simulink model "Trajectory_closest_point_info_get"  (R2021a)
settings: configuration reference "AION_IDS_Speedgoat" (kept outside this file)
undefined symbols (not defined in the file): CLOSEST_DISTANCE_THRESHOLD, DEG2RAD, DELTA_ANGLE_COMPENSATION1, DELTA_ANGLE_COMPENSATION2, DELTA_ANGLE_DIVISOR360, DELTA_ANGLE_THRESHOLD, N_ALTERNATIVE_CLOSEST_POINT_QUEUE, SINGLE_STEP_MOTION_ARC_LENGTH_THRESHOLD
libraries: simulink x7
(part 1 of 2)
Description:
  | 获取参考轨迹中的最近点信息
settings Model: DataDictionary=Trajectory_Closest_Point_Info_Get.sldd  Creator=xinrui  LastModifiedBy=Administrator
settings ConfigSetRef: SourceName=AION_IDS_Speedgoat

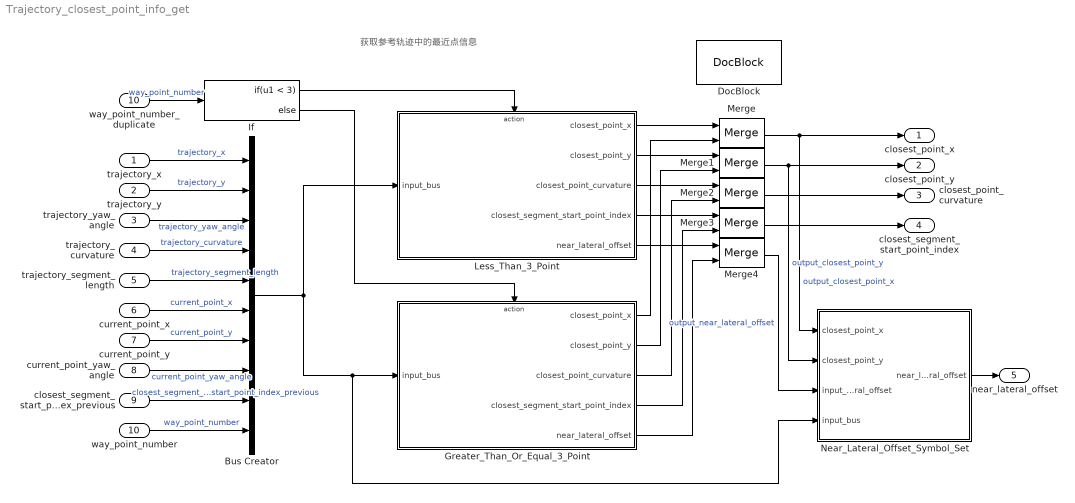
== system Trajectory_closest_point_info_get ==
  note: 获取参考轨迹中的最近点信息
  trajectory_x : Inport  Description=参考轨迹的x坐标序列，实数，m。  OutDataTypeStr=double  PortDimensions=MAX_GLOBAL_TRAJECTORY_WAY_POINT_NUMBER  Interpolate=off
  trajectory_y : Inport  Description=参考轨迹的y坐标序列，实数，m。  Port=2  OutDataTypeStr=double  PortDimensions=MAX_GLOBAL_TRAJECTORY_WAY_POINT_NUMBER  Interpolate=off
  trajectory_yaw_angle : Inport  Description=参考轨迹横摆角序列，实数，deg。  Port=3  OutDataTypeStr=double  PortDimensions=MAX_GLOBAL_TRAJECTORY_WAY_POINT_NUMBER  Interpolate=off
  trajectory_curvature : Inport  Description=参考轨迹曲率序列，实数，1/m。  Port=4  OutDataTypeStr=double  PortDimensions=MAX_GLOBAL_TRAJECTORY_WAY_POINT_NUMBER  Interpolate=off
  trajectory_segment_length : Inport  Description=参考轨迹相邻两点之间的线段长度序列，实数，m。  Port=5  OutDataTypeStr=double  PortDimensions=MAX_GLOBAL_TRAJECTORY_WAY_POINT_NUMBER  Interpolate=off
  current_point_x : Inport  Description=车辆所处的当前点x坐标，实数，m。  Port=6  OutDataTypeStr=double  Interpolate=off
  current_point_y : Inport  Description=车辆所处的当前点y坐标，实数，m。  Port=7  OutDataTypeStr=double  Interpolate=off
  current_point_yaw_angle : Inport  Description=当前车辆横摆角，实数，deg。  Port=8  OutDataTypeStr=double  Interpolate=off
  closest_segment_start_point_index_previous : Inport  Description=上周期最近路点线段起始点索引（从1开始计数），自然数，无量纲。  Port=9  OutDataTypeStr=int32  Interpolate=off
  way_point_number : Inport  Description=参考轨迹路点数量，自然数，无量纲。  Port=10  OutDataTypeStr=int32  Interpolate=off
  Bus Creator : BusCreator  Inputs=10
  DocBlock : simulink/Model-Wide Utilities/DocBlock  DocumentType=HTML  mask(DocBlock){}
      mask Display:
      | plot([.8 0 0 1 1 .8 .8 1],[1 1 0 0 .8 1 .8 .8]);
      | text(.5,.6,'CHANGELOG','horizontalalignment','center');
      | text(.95,.05,get_param(gcb,'DocumentType'),'verticalalignment','bottom','horizontalalignment','right');
  Greater_Than_Or_Equal_3_Point : Subsystem  Description=参考轨迹路点数大于等于3个时，采用局部搜索或者全局搜索获取最近点。  TreatAsAtomicUnit=on
  If : If  Description=|  IfExpression=u1 < 3
      | （1）参考轨迹路点数少于3个时使用倒数2个点进行向量投影，获取最近点。
      | （2）参考轨迹路点数大于等于3个时，采用局部搜索或者全局搜索获取最近点。
  Less_Than_3_Point : Subsystem  Description=参考轨迹路点数少于3个时使用倒数2个点进行向量投影，获取最近点。  TreatAsAtomicUnit=on
  Merge{,1..4} (5 alike) : Merge
  Near_Lateral_Offset_Symbol_Set : Subsystem  Description=设置最近处横向偏差的正负符号。
  way_point_number_duplicate : InportShadow  Description=第二个点的x坐标。  Port=10  OutDataTypeStr=int32  Interpolate=off
  closest_point_x : Outport  Description=最近点x坐标，实数，m。  OutDataTypeStr=double
  closest_point_y : Outport  Description=最近点y坐标，实数，m。  Port=2  OutDataTypeStr=double
  closest_point_curvature : Outport  Description=最近点曲率，实数，1/m。  Port=3  OutDataTypeStr=double
  closest_segment_start_point_index : Outport  Description=最近路点线段起始点索引（从1开始计数），自然数，无量纲。  Port=4  OutDataTypeStr=int32
  near_lateral_offset : Outport  Description=最近处横向偏差，实数，m。  Port=5  OutDataTypeStr=double
  wires:
  trajectory_x/1 -> Bus Creator/1  "trajectory_x"
  trajectory_y/1 -> Bus Creator/2  "trajectory_y"
  trajectory_yaw_angle/1 -> Bus Creator/3  "trajectory_yaw_angle"
  trajectory_curvature/1 -> Bus Creator/4  "trajectory_curvature"
  trajectory_segment_length/1 -> Bus Creator/5  "trajectory_segment_length"
  current_point_x/1 -> Bus Creator/6  "current_point_x"
  current_point_y/1 -> Bus Creator/7  "current_point_y"
  current_point_yaw_angle/1 -> Bus Creator/8  "current_point_yaw_angle"
  closest_segment_start_point_index_previous/1 -> Bus Creator/9  "closest_segment_start_point_index_previous"
  way_point_number/1 -> Bus Creator/10  "way_point_number"
  If/1 -> Less_Than_3_Point/Action
  way_point_number_duplicate/1 -> If/1  "way_point_number"
  Bus Creator/1 -> Less_Than_3_Point/1(input_bus), Near_Lateral_Offset_Symbol_Set/4(input_bus), Greater_Than_Or_Equal_3_Point/1(input_bus)
  If/2 -> Greater_Than_Or_Equal_3_Point/Action
  Greater_Than_Or_Equal_3_Point/1(closest_point_x) -> Merge/2
  Less_Than_3_Point/1(closest_point_x) -> Merge/1
  Less_Than_3_Point/2(closest_point_y) -> Merge1/1
  Greater_Than_Or_Equal_3_Point/2(closest_point_y) -> Merge1/2
  Less_Than_3_Point/3(closest_point_curvature) -> Merge2/1
  Greater_Than_Or_Equal_3_Point/3(closest_point_curvature) -> Merge2/2
  Less_Than_3_Point/4(closest_segment_start_point_index) -> Merge3/1
  Greater_Than_Or_Equal_3_Point/4(closest_segment_start_point_index) -> Merge3/2
  Less_Than_3_Point/5(near_lateral_offset) -> Merge4/1
  Greater_Than_Or_Equal_3_Point/5(near_lateral_offset) -> Merge4/2
  Merge1/1 -> closest_point_y/1, Near_Lateral_Offset_Symbol_Set/2(closest_point_y)  "output_closest_point_y"
  Merge2/1 -> closest_point_curvature/1
  Merge3/1 -> closest_segment_start_point_index/1
  Merge/1 -> closest_point_x/1, Near_Lateral_Offset_Symbol_Set/1(closest_point_x)  "output_closest_point_x"
  Near_Lateral_Offset_Symbol_Set/1(near_lateral_offset) -> near_lateral_offset/1
  Merge4/1 -> Near_Lateral_Offset_Symbol_Set/3(input_near_lateral_offset)  "output_near_lateral_offset"

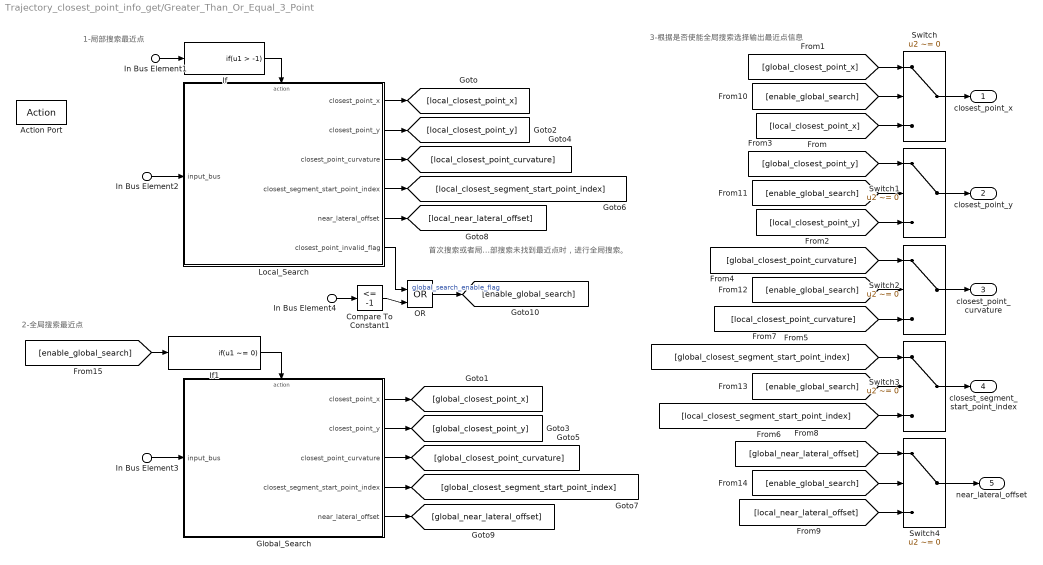
== system Trajectory_closest_point_info_get/Greater_Than_Or_Equal_3_Point ==
  note: 首次搜索或者局部搜索未找到最近点时，进行全局搜索。
  note: 3-根据是否使能全局搜索选择输出最近点信息
  note: 2-全局搜索最近点
  note: 1-局部搜索最近点
  In Bus Element2 : Inport  PortName=input_bus
  In Bus Element3 : Inport  PortName=input_bus
  In Bus Element1 : Inport  PortName=input_bus  Element=closest_segment_start_point_index_previous
  In Bus Element4 : Inport  PortName=input_bus  Element=closest_segment_start_point_index_previous
  Action Port : ActionPort  PropagateVarSize=During execution  ActionPortLabel=else
  Compare To Constant1 : simulink/Logic and Bit Operations/Compare To Constant  Description=如果上周期最近线段起始点索引小于等于-1，代表首次搜索，开启全局搜索。  relop=<=  const=-1  OutDataTypeStr=boolean
  Global_Search : Subsystem  Description=首次搜索或者局部搜索未找到最近点时，进行全局搜索。  TreatAsAtomicUnit=on
  If : If  Description=上周期最近路点线段起始点索引大于-1时，说明上周期找到了最近点，本周期可以采用局部搜索获取最近点。  IfExpression=u1 > -1  ShowElse=off
  If1 : If  Description=首次搜索或者局部搜索未找到最近点时，进行全局搜索。  IfExpression=u1 ~= 0  ShowElse=off
  Local_Search : Subsystem  Description=非首次搜索采用上周期最近路点线段起始点前后各1.11m范围（按最高车速80km/h换算到50ms）进行局部搜索。  TreatAsAtomicUnit=on
  OR : Logic  Description=首次搜索或者局部搜索未找到最近点时，进行全局搜索。  Operator=OR  IconShape=distinctive  AllPortsSameDT=off  OutDataTypeStr=boolean
  Switch{,1..4} (5 alike) : Switch  Criteria=u2 ~= 0
  closest_point_x : Outport  Description=最近点x坐标，实数，m。  OutDataTypeStr=double
  closest_point_y : Outport  Description=最近点y坐标，实数，m。  Port=2  OutDataTypeStr=double
  closest_point_curvature : Outport  Description=最近点曲率，实数，1/m。  Port=3  OutDataTypeStr=double
  closest_segment_start_point_index : Outport  Description=最近路点线段起始点索引，自然数，无量纲。  Port=4  OutDataTypeStr=int32
  near_lateral_offset : Outport  Description=最近处横向偏差，实数，m。  Port=5  OutDataTypeStr=double
  wires:
  In Bus Element2/1 -> Local_Search/1(input_bus)
  If/1 -> Local_Search/Action
  In Bus Element1/1 -> If/1
  In Bus Element3/1 -> Global_Search/1(input_bus)
  In Bus Element4/1 -> Compare To Constant1/1
  If1/1 -> Global_Search/Action
  OR/1 -> [enable_global_search]  "global_search_enable_flag"
  Switch/1 -> closest_point_x/1
  Switch1/1 -> closest_point_y/1
  Switch2/1 -> closest_point_curvature/1
  Switch3/1 -> closest_segment_start_point_index/1
  Switch4/1 -> near_lateral_offset/1
  Local_Search/1(closest_point_x) -> [local_closest_point_x]
  Global_Search/1(closest_point_x) -> [global_closest_point_x]
  [global_closest_point_x] -> Switch/1
  [local_closest_point_x] -> Switch/3
  Local_Search/2(closest_point_y) -> [local_closest_point_y]
  Global_Search/2(closest_point_y) -> [global_closest_point_y]
  [global_closest_point_y] -> Switch1/1
  [local_closest_point_y] -> Switch1/3
  Local_Search/3(closest_point_curvature) -> [local_closest_point_curvature]
  Global_Search/3(closest_point_curvature) -> [global_closest_point_curvature]
  [global_closest_point_curvature] -> Switch2/1
  [local_closest_point_curvature] -> Switch2/3
  Local_Search/4(closest_segment_start_point_index) -> [local_closest_segment_start_point_index]
  Global_Search/4(closest_segment_start_point_index) -> [global_closest_segment_start_point_index]
  [global_closest_segment_start_point_index] -> Switch3/1
  [local_closest_segment_start_point_index] -> Switch3/3
  Local_Search/5(near_lateral_offset) -> [local_near_lateral_offset]
  Global_Search/5(near_lateral_offset) -> [global_near_lateral_offset]
  [local_near_lateral_offset] -> Switch4/3
  [global_near_lateral_offset] -> Switch4/1
  [enable_global_search] -> Switch/2
  [enable_global_search] -> Switch1/2
  [enable_global_search] -> Switch2/2
  [enable_global_search] -> Switch3/2
  [enable_global_search] -> Switch4/2
  Compare To Constant1/1 -> OR/2
  Local_Search/6(closest_point_invalid_flag) -> OR/1
  [enable_global_search] -> If1/1

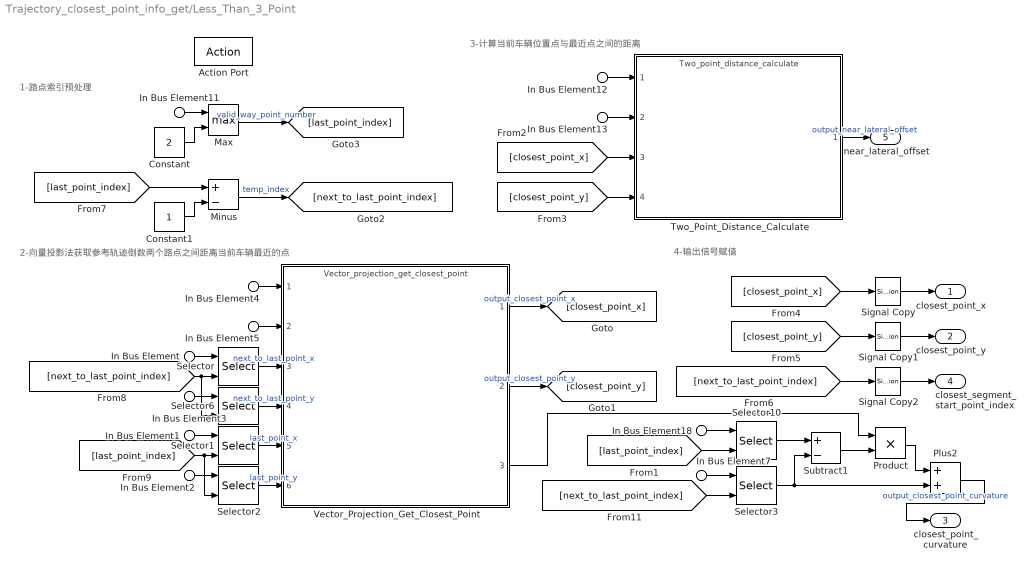
== system Trajectory_closest_point_info_get/Less_Than_3_Point ==
  note: 4-输出信号赋值
  note: 3-计算当前车辆位置点与最近点之间的距离
  note: 2-向量投影法获取参考轨迹倒数两个路点之间距离当前车辆最近的点
  note: 1-路点索引预处理
  In Bus Element7 : Inport  PortName=input_bus  Element=trajectory_curvature
  In Bus Element18 : Inport  PortName=input_bus  Element=trajectory_curvature
  In Bus Element4 : Inport  PortName=input_bus  Element=current_point_x
  In Bus Element12 : Inport  PortName=input_bus  Element=current_point_x
  In Bus Element5 : Inport  PortName=input_bus  Element=current_point_y
  In Bus Element13 : Inport  PortName=input_bus  Element=current_point_y
  In Bus Element11 : Inport  PortName=input_bus  Element=way_point_number
  In Bus Element : Inport  PortName=input_bus  Element=trajectory_x
  In Bus Element1 : Inport  PortName=input_bus  Element=trajectory_x
  In Bus Element3 : Inport  PortName=input_bus  Element=trajectory_y
  In Bus Element2 : Inport  PortName=input_bus  Element=trajectory_y
  Action Port : ActionPort  InitializeStates=reset  PropagateVarSize=During execution  ActionPortLabel=if(u1 < 3)
  Constant : Constant  Value=2  OutDataTypeStr=int32  SampleTime=-1
  Constant1 : Constant  OutDataTypeStr=int32  SampleTime=-1
  Max : MinMax  Description=参考轨迹路点数量不得少于2，获取最大路点数量，减一即为倒数第一个路点索引。  Function=max  Inputs=2  OutDataTypeStr=int32
  Minus : Sum  Description=计算参考轨迹上倒数第二个点的索引。  Inputs=+-
  Plus2 : Sum  Description=根据线段起始点、结束点的曲率线性插值得到最近点的曲率。
  Product : Product  Description=按比例计算线段起始点到最近点的曲率增量。
  Selector : Selector  Description=获取参考轨迹倒数第二个路点的x坐标。  IndexOptions=Index vector (port)  Indices=[1 3]  OutputSizes=1
  Selector1 : Selector  Description=获取参考轨迹最后一个路点的x坐标。  IndexOptions=Index vector (port)  Indices=[1 3]  OutputSizes=1
  Selector10 : Selector  Description=获取当前遍历路点的下一个路点的曲率。  IndexOptions=Index vector (port)  Indices=[1 3]  OutputSizes=1
  Selector2 : Selector  Description=获取参考轨迹最后一个路点的y坐标。  IndexOptions=Index vector (port)  Indices=[1 3]  OutputSizes=1
  Selector3 : Selector  Description=获取当前遍历路点的曲率。  IndexOptions=Index vector (port)  Indices=[1 3]  OutputSizes=1
  Selector6 : Selector  Description=获取参考轨迹倒数第二个路点的y坐标。  IndexOptions=Index vector (port)  Indices=[1 3]  OutputSizes=1
  Signal Copy : SignalConversion  OverrideOpt=off
  Signal Copy1 : SignalConversion  OverrideOpt=off
  Signal Copy2 : SignalConversion  OverrideOpt=off
  Subtract1 : Sum  Description=计算线段起始点到结束点的曲率增量。  Inputs=+-
  Two_Point_Distance_Calculate : ModelReference  Description=计算车辆当前点与参考轨迹上的最近点之间的距离。  ModelNameDialog=Two_point_distance_calculate.slx  SimulationMode=Normal  ModelReferenceVersion=4.61
  Vector_Projection_Get_Closest_Point : ModelReference  Description=向量投影法获取最近点。  ModelNameDialog=Vector_projection_get_closest_point.slx  SimulationMode=Normal  ModelReferenceVersion=4.54
  closest_point_x : Outport  Description=最近点x坐标，实数，m。  OutDataTypeStr=double
  closest_point_y : Outport  Description=最近点y坐标，实数，m。  Port=2  OutDataTypeStr=double
  closest_point_curvature : Outport  Description=最近点曲率，实数，1/m。  Port=3  OutDataTypeStr=double
  closest_segment_start_point_index : Outport  Description=最近路点线段起始点索引，自然数，无量纲。  Port=4  OutDataTypeStr=int32
  near_lateral_offset : Outport  Description=最近处横向偏差，实数，m。  Port=5  OutDataTypeStr=double
  wires:
  In Bus Element1/1 -> Selector1/1
  In Bus Element11/1 -> Max/1
  In Bus Element5/1 -> Vector_Projection_Get_Closest_Point/2
  [last_point_index] -> Selector2/2, Selector1/2
  Plus2/1 -> closest_point_curvature/1  "output_closest_point_curvature"
  Two_Point_Distance_Calculate/1 -> near_lateral_offset/1  "output_near_lateral_offset"
  Selector1/1 -> Vector_Projection_Get_Closest_Point/5  "last_point_x"
  Vector_Projection_Get_Closest_Point/1 -> [closest_point_x]  "output_closest_point_x"
  Selector2/1 -> Vector_Projection_Get_Closest_Point/6  "last_point_y"
  [next_to_last_point_index] -> Signal Copy2/1
  [last_point_index] -> Minus/1
  In Bus Element3/1 -> Selector6/1
  Selector6/1 -> Vector_Projection_Get_Closest_Point/4  "next_to_last_point_y"
  [next_to_last_point_index] -> Selector6/2, Selector/2
  Constant/1 -> Max/2
  In Bus Element2/1 -> Selector2/1
  In Bus Element/1 -> Selector/1
  Selector/1 -> Vector_Projection_Get_Closest_Point/3  "next_to_last_point_x"
  Vector_Projection_Get_Closest_Point/3 -> Product/1
  Minus/1 -> [next_to_last_point_index]  "temp_index"
  Vector_Projection_Get_Closest_Point/2 -> [closest_point_y]  "output_closest_point_y"
  In Bus Element4/1 -> Vector_Projection_Get_Closest_Point/1
  [closest_point_y] -> Signal Copy1/1
  Max/1 -> [last_point_index]  "valid_way_point_number"
  Constant1/1 -> Minus/2
  [closest_point_x] -> Signal Copy/1
  [closest_point_x] -> Two_Point_Distance_Calculate/3
  [closest_point_y] -> Two_Point_Distance_Calculate/4
  In Bus Element12/1 -> Two_Point_Distance_Calculate/1
  In Bus Element13/1 -> Two_Point_Distance_Calculate/2
  [last_point_index] -> Selector10/2
  In Bus Element18/1 -> Selector10/1
  In Bus Element7/1 -> Selector3/1
  [next_to_last_point_index] -> Selector3/2
  Product/1 -> Plus2/1
  Selector3/1 -> Subtract1/2, Plus2/2
  Subtract1/1 -> Product/2
  Selector10/1 -> Subtract1/1
  Signal Copy/1 -> closest_point_x/1
  Signal Copy1/1 -> closest_point_y/1
  Signal Copy2/1 -> closest_segment_start_point_index/1

== system Trajectory_closest_point_info_get/Near_Lateral_Offset_Symbol_Set ==
  note: 车辆与参考轨迹最近处横向偏差的符号和最近点在车辆坐标系下的y坐标符号相同。
  closest_point_x : Inport  Description=最近点x坐标，实数，m。  OutDataTypeStr=double
  closest_point_y : Inport  Description=最近点y坐标，实数，m。  Port=2  OutDataTypeStr=double
  input_near_lateral_offset : Inport  Description=输入的原始最近处横向偏差绝对值，正实数，m。  Port=3  OutDataTypeStr=double
  In Bus Element10 : Inport  Port=4  PortName=input_bus  Element=current_point_yaw_angle
  In Bus Element8 : Inport  Port=4  PortName=input_bus  Element=current_point_x
  In Bus Element9 : Inport  Port=4  PortName=input_bus  Element=current_point_y
  Multiply : Gain  Description=将以度为单位的当前车辆横摆角换算为弧度单位，以便输入给车辆坐标系转换模型。  Gain=DEG2RAD
  Switch : Switch  Description=车辆与参考轨迹最近处横向偏差的符号和最近点在车辆坐标系下的y坐标符号相同。
  Terminator : Terminator
  Unary Minus : UnaryMinus  Description=对近处横向偏差数值取负号。
  Vehicle_Coordinate_Transfer : ModelReference  Description=将参考轨迹上的最近点转换到车辆坐标系下。  ModelNameDialog=Vehicle_coordinate_transfer.slx  SimulationMode=Normal  ModelReferenceVersion=4.54
  near_lateral_offset : Outport  Description=最近处横向偏差，实数，m。  OutDataTypeStr=double
  wires:
  In Bus Element9/1 -> Vehicle_Coordinate_Transfer/2
  closest_point_y/1 -> Vehicle_Coordinate_Transfer/4
  closest_point_x/1 -> Vehicle_Coordinate_Transfer/3
  In Bus Element8/1 -> Vehicle_Coordinate_Transfer/1
  In Bus Element10/1 -> Multiply/1
  Multiply/1 -> Vehicle_Coordinate_Transfer/5  "yaw_angle_rad"
  Vehicle_Coordinate_Transfer/2 -> Switch/2  "vehicle_y1"
  Vehicle_Coordinate_Transfer/1 -> Terminator/1  "vehicle_x1"
  input_near_lateral_offset/1 -> Switch/1, Unary Minus/1
  Unary Minus/1 -> Switch/3
  Switch/1 -> near_lateral_offset/1  "output_near_lateral_offset"

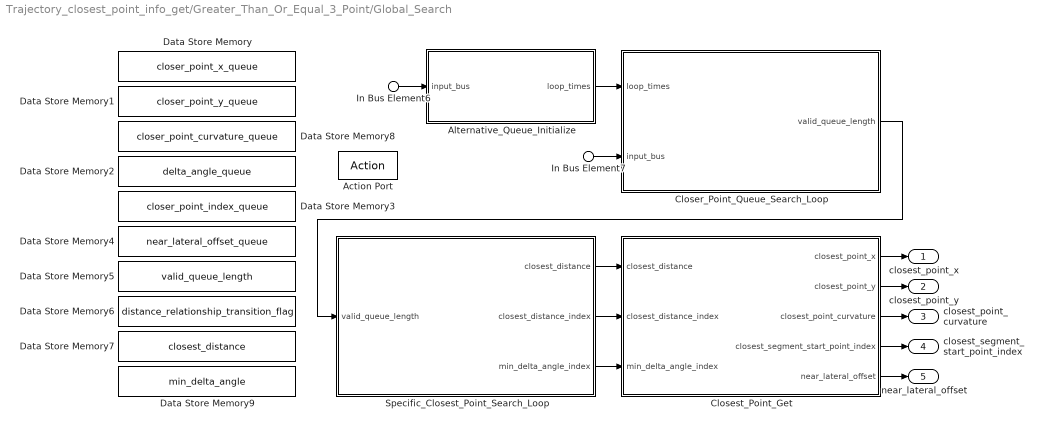
== system Trajectory_closest_point_info_get/Greater_Than_Or_Equal_3_Point/Global_Search ==
  In Bus Element6 : Inport  PortName=input_bus
  In Bus Element7 : Inport  PortName=input_bus
  Action Port : ActionPort  InitializeStates=reset  PropagateVarSize=During execution  ActionPortLabel=if(u1 ~= 0)
  Alternative_Queue_Initialize : Subsystem  Description=备选最近点序列初始化。
  Closer_Point_Queue_Search_Loop : Subsystem  Description=遍历搜索备选最近点序列信息。  TreatAsAtomicUnit=on
  Closest_Point_Get : Subsystem  Description=提取最近点。
  Data Store Memory : DataStoreMemory  DataStoreName=closer_point_x_queue  ReadBeforeWriteMsg=warning  WriteAfterWriteMsg=warning  WriteAfterReadMsg=warning  InitialValue=zeros(N_ALTERNATIVE_CLOSEST_POINT_QUEUE, 1)  VectorParams1D=off  ShowAdditionalParam=off  OutDataTypeStr=double  StateMustResolveToSignalObject=on
  Data Store Memory1 : DataStoreMemory  DataStoreName=closer_point_y_queue  ReadBeforeWriteMsg=warning  WriteAfterWriteMsg=warning  WriteAfterReadMsg=warning  InitialValue=zeros(N_ALTERNATIVE_CLOSEST_POINT_QUEUE, 1)  VectorParams1D=off  ShowAdditionalParam=off  OutDataTypeStr=double  StateMustResolveToSignalObject=on
  Data Store Memory2 : DataStoreMemory  DataStoreName=delta_angle_queue  ReadBeforeWriteMsg=warning  WriteAfterWriteMsg=warning  WriteAfterReadMsg=warning  InitialValue=zeros(N_ALTERNATIVE_CLOSEST_POINT_QUEUE, 1)  VectorParams1D=off  ShowAdditionalParam=off  OutDataTypeStr=double  StateMustResolveToSignalObject=on
  Data Store Memory3 : DataStoreMemory  DataStoreName=closer_point_index_queue  ReadBeforeWriteMsg=warning  WriteAfterWriteMsg=warning  WriteAfterReadMsg=warning  InitialValue=zeros(N_ALTERNATIVE_CLOSEST_POINT_QUEUE, 1)  VectorParams1D=off  ShowAdditionalParam=off  OutDataTypeStr=int32  StateMustResolveToSignalObject=on
  Data Store Memory4 : DataStoreMemory  DataStoreName=near_lateral_offset_queue  ReadBeforeWriteMsg=warning  WriteAfterWriteMsg=warning  WriteAfterReadMsg=warning  InitialValue=zeros(N_ALTERNATIVE_CLOSEST_POINT_QUEUE, 1)  VectorParams1D=off  ShowAdditionalParam=off  OutDataTypeStr=double  StateMustResolveToSignalObject=on
  Data Store Memory5 : DataStoreMemory  DataStoreName=valid_queue_length  ReadBeforeWriteMsg=warning  WriteAfterWriteMsg=warning  WriteAfterReadMsg=warning  VectorParams1D=off  ShowAdditionalParam=off  OutDataTypeStr=int32  StateMustResolveToSignalObject=on
  Data Store Memory6 : DataStoreMemory  DataStoreName=distance_relationship_transition_flag  ReadBeforeWriteMsg=warning  WriteAfterWriteMsg=warning  WriteAfterReadMsg=warning  VectorParams1D=off  ShowAdditionalParam=off  OutDataTypeStr=boolean  StateMustResolveToSignalObject=on
  Data Store Memory7 : DataStoreMemory  DataStoreName=closest_distance  ReadBeforeWriteMsg=warning  WriteAfterWriteMsg=warning  WriteAfterReadMsg=warning  VectorParams1D=off  ShowAdditionalParam=off  OutDataTypeStr=double  StateMustResolveToSignalObject=on
  Data Store Memory8 : DataStoreMemory  DataStoreName=closer_point_curvature_queue  ReadBeforeWriteMsg=warning  WriteAfterWriteMsg=warning  WriteAfterReadMsg=warning  InitialValue=zeros(N_ALTERNATIVE_CLOSEST_POINT_QUEUE, 1)  VectorParams1D=off  ShowAdditionalParam=off  OutDataTypeStr=double  StateMustResolveToSignalObject=on
  Data Store Memory9 : DataStoreMemory  DataStoreName=min_delta_angle  ReadBeforeWriteMsg=warning  WriteAfterWriteMsg=warning  WriteAfterReadMsg=warning  VectorParams1D=off  ShowAdditionalParam=off  OutDataTypeStr=double  StateMustResolveToSignalObject=on
  Specific_Closest_Point_Search_Loop : Subsystem  Description=|  TreatAsAtomicUnit=on
      | 遍历备选最近点序列，找到如下两种路点：
      | （1）与本车距离最近的点。
      | （2）与本车距离小于阈值且横摆夹角最小的点。
  closest_point_x : Outport  Description=最近点x坐标，实数，m。  OutDataTypeStr=double
  closest_point_y : Outport  Description=最近点y坐标，实数，m。  Port=2  OutDataTypeStr=double
  closest_point_curvature : Outport  Description=最近点曲率，实数，1/m。  Port=3  OutDataTypeStr=double
  closest_segment_start_point_index : Outport  Description=最近路点线段起始点索引，自然数，无量纲。  Port=4  OutDataTypeStr=int32
  near_lateral_offset : Outport  Description=最近处横向偏差，实数，m。  Port=5  OutDataTypeStr=double
  wires:
  In Bus Element6/1 -> Alternative_Queue_Initialize/1(input_bus)
  In Bus Element7/1 -> Closer_Point_Queue_Search_Loop/2(input_bus)
  Alternative_Queue_Initialize/1(loop_times) -> Closer_Point_Queue_Search_Loop/1(loop_times)
  Closer_Point_Queue_Search_Loop/1(valid_queue_length) -> Specific_Closest_Point_Search_Loop/1(valid_queue_length)
  Specific_Closest_Point_Search_Loop/2(closest_distance_index) -> Closest_Point_Get/2(closest_distance_index)
  Specific_Closest_Point_Search_Loop/3(min_delta_angle_index) -> Closest_Point_Get/3(min_delta_angle_index)
  Closest_Point_Get/1(closest_point_x) -> closest_point_x/1
  Closest_Point_Get/2(closest_point_y) -> closest_point_y/1
  Closest_Point_Get/3(closest_point_curvature) -> closest_point_curvature/1
  Closest_Point_Get/4(closest_segment_start_point_index) -> closest_segment_start_point_index/1
  Closest_Point_Get/5(near_lateral_offset) -> near_lateral_offset/1
  Specific_Closest_Point_Search_Loop/1(closest_distance) -> Closest_Point_Get/1(closest_distance)

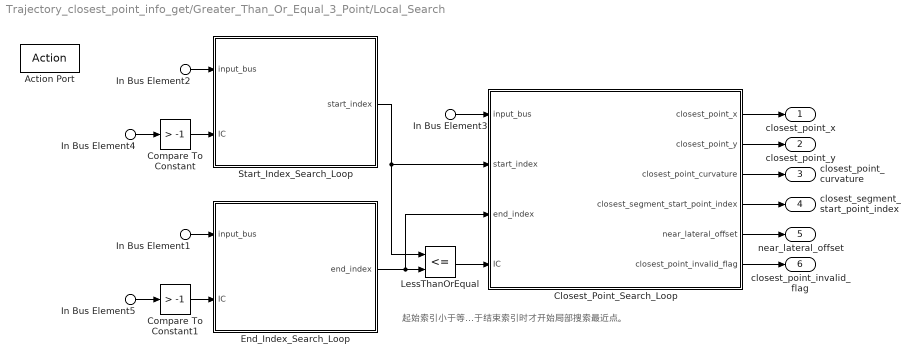
== system Trajectory_closest_point_info_get/Greater_Than_Or_Equal_3_Point/Local_Search ==
  note: 起始索引小于等于结束索引时才开始局部搜索最近点。
  In Bus Element2 : Inport  PortName=input_bus
  In Bus Element1 : Inport  PortName=input_bus
  In Bus Element3 : Inport  PortName=input_bus
  In Bus Element4 : Inport  PortName=input_bus  Element=closest_segment_start_point_index_previous
  In Bus Element5 : Inport  PortName=input_bus  Element=closest_segment_start_point_index_previous
  Action Port : ActionPort  InitializeStates=reset  PropagateVarSize=During execution  ActionPortLabel=if(u1 > -1)
  Closest_Point_Search_Loop : Subsystem  Description=搜索上一个周期最近点索引前后1.11m范围（按最高80km/h车速）内的本周期最近点信息。  TreatAsAtomicUnit=on
  Compare To Constant : simulink/Logic and Bit Operations/Compare To Constant  Description=确认上周期最近线段起始点索引大于-1，代表非首次搜索，才开启局部起始点搜索。  relop=>  const=-1  OutDataTypeStr=boolean
  Compare To Constant1 : simulink/Logic and Bit Operations/Compare To Constant  Description=确认上周期最近线段起始点索引大于-1，代表非首次搜索，才开启局部结束点搜索。  relop=>  const=-1  OutDataTypeStr=boolean
  End_Index_Search_Loop : Subsystem  Description=搜索上一个周期最近点索引后1.11m范围（按最高80km/h车速）的结束索引。  TreatAsAtomicUnit=on
  LessThanOrEqual : RelationalOperator  Description=起始索引小于等于结束索引时才开始局部搜索最近点。  Operator=<=  OutDataTypeStr=boolean  RndMeth=Simplest
  Start_Index_Search_Loop : Subsystem  Description=搜索上一个周期最近点索引前1.11m范围（按最高80km/h车速）的起始索引。  TreatAsAtomicUnit=on
  closest_point_x : Outport  Description=最近点x坐标，实数，m。  OutDataTypeStr=double
  closest_point_y : Outport  Description=最近点y坐标，实数，m。  Port=2  OutDataTypeStr=double
  closest_point_curvature : Outport  Description=最近点曲率，实数，1/m。  Port=3  OutDataTypeStr=double
  closest_segment_start_point_index : Outport  Description=最近路点线段起始点索引，自然数，无量纲。  Port=4  OutDataTypeStr=int32
  near_lateral_offset : Outport  Description=最近处横向偏差，实数，m。  Port=5  OutDataTypeStr=double
  closest_point_invalid_flag : Outport  Description=最近点有效标志。  Port=6  OutDataTypeStr=boolean
  wires:
  In Bus Element4/1 -> Compare To Constant/1
  In Bus Element5/1 -> Compare To Constant1/1
  In Bus Element2/1 -> Start_Index_Search_Loop/1(input_bus)
  In Bus Element1/1 -> End_Index_Search_Loop/1(input_bus)
  In Bus Element3/1 -> Closest_Point_Search_Loop/1(input_bus)
  LessThanOrEqual/1 -> Closest_Point_Search_Loop/4(IC)
  Start_Index_Search_Loop/1(start_index) -> Closest_Point_Search_Loop/2(start_index), LessThanOrEqual/1
  End_Index_Search_Loop/1(end_index) -> Closest_Point_Search_Loop/3(end_index), LessThanOrEqual/2
  Compare To Constant/1 -> Start_Index_Search_Loop/2(IC)
  Compare To Constant1/1 -> End_Index_Search_Loop/2(IC)
  Closest_Point_Search_Loop/1(closest_point_x) -> closest_point_x/1
  Closest_Point_Search_Loop/2(closest_point_y) -> closest_point_y/1
  Closest_Point_Search_Loop/3(closest_point_curvature) -> closest_point_curvature/1
  Closest_Point_Search_Loop/4(closest_segment_start_point_index) -> closest_segment_start_point_index/1
  Closest_Point_Search_Loop/5(near_lateral_offset) -> near_lateral_offset/1
  Closest_Point_Search_Loop/6(closest_point_invalid_flag) -> closest_point_invalid_flag/1

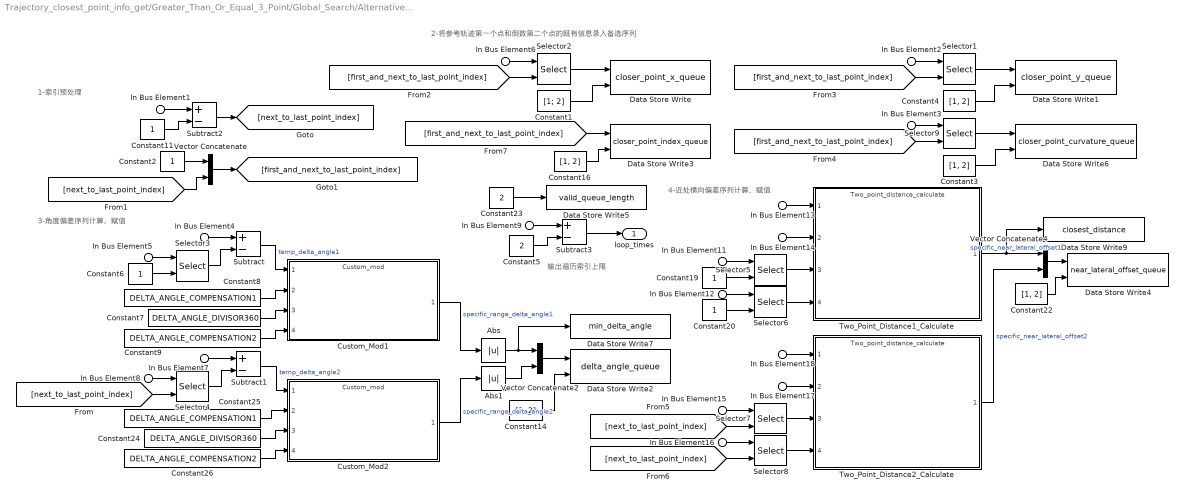
== system Trajectory_closest_point_info_get/Greater_Than_Or_Equal_3_Point/Global_Search/Alternative_Queue_Initialize ==
  note: 输出遍历索引上限
  note: 4-近处横向偏差序列计算、赋值
  note: 3-角度偏差序列计算、赋值
  note: 2-将参考轨迹第一个点和倒数第二个点的既有信息录入备选序列
  note: 1-索引预处理
  In Bus Element6 : Inport  PortName=input_bus  Element=trajectory_x
  In Bus Element11 : Inport  PortName=input_bus  Element=trajectory_x
  In Bus Element15 : Inport  PortName=input_bus  Element=trajectory_x
  In Bus Element1 : Inport  PortName=input_bus  Element=way_point_number
  In Bus Element9 : Inport  PortName=input_bus  Element=way_point_number
  In Bus Element2 : Inport  PortName=input_bus  Element=trajectory_y
  In Bus Element12 : Inport  PortName=input_bus  Element=trajectory_y
  In Bus Element16 : Inport  PortName=input_bus  Element=trajectory_y
  In Bus Element4 : Inport  PortName=input_bus  Element=current_point_yaw_angle
  In Bus Element7 : Inport  PortName=input_bus  Element=current_point_yaw_angle
  In Bus Element5 : Inport  PortName=input_bus  Element=trajectory_yaw_angle
  In Bus Element8 : Inport  PortName=input_bus  Element=trajectory_yaw_angle
  In Bus Element14 : Inport  PortName=input_bus  Element=current_point_y
  In Bus Element17 : Inport  PortName=input_bus  Element=current_point_y
  In Bus Element13 : Inport  PortName=input_bus  Element=current_point_x
  In Bus Element18 : Inport  PortName=input_bus  Element=current_point_x
  In Bus Element3 : Inport  PortName=input_bus  Element=trajectory_curvature
  Abs : Abs
  Abs1 : Abs
  Constant1 : Constant  Value=[1; 2]  OutDataTypeStr=int32  SampleTime=-1
  Constant{2,6,11,19..20} (5 alike) : Constant  OutDataTypeStr=int32  SampleTime=-1
  Constant{3..4,14,16,22} (5 alike) : Constant  Value=[1, 2]  OutDataTypeStr=int32  SampleTime=-1
  Constant23 : Constant  Value=2  OutDataTypeStr=int32  SampleTime=-1
  Constant24 : Constant  Value=DELTA_ANGLE_DIVISOR360  OutDataTypeStr=double  SampleTime=-1
  Constant25 : Constant  Value=DELTA_ANGLE_COMPENSATION1  OutDataTypeStr=double  SampleTime=-1
  Constant26 : Constant  Value=DELTA_ANGLE_COMPENSATION2  OutDataTypeStr=double  SampleTime=-1
  Constant5 : Constant  Value=2  OutDataTypeStr=int32  SampleTime=-1
  Constant7 : Constant  Value=DELTA_ANGLE_DIVISOR360  OutDataTypeStr=double  SampleTime=-1
  Constant8 : Constant  Value=DELTA_ANGLE_COMPENSATION1  OutDataTypeStr=double  SampleTime=-1
  Constant9 : Constant  Value=DELTA_ANGLE_COMPENSATION2  OutDataTypeStr=double  SampleTime=-1
  Custom_Mod1 : ModelReference  Description=对当前车辆横摆角与参考轨迹起点横摆角偏差取模到-180~180度范围内。  ModelNameDialog=Custom_mod  SimulationMode=Normal  ModelReferenceVersion=4.78
  Custom_Mod2 : ModelReference  Description=对当前车辆横摆角与参考轨迹倒数第二个点横摆角偏差取模到-180~180度范围内。  ModelNameDialog=Custom_mod  SimulationMode=Normal  ModelReferenceVersion=4.78
  Data Store Write : DataStoreWrite  DataStoreName=closer_point_x_queue  DataStoreElements=closer_point_x_queue  EnableIndexing=on  NumberOfDimensions=2  IndexOptions=Index vector (port),Index vector (dialog)  Indices=1,1  OutputSizes=1,1
  Data Store Write1 : DataStoreWrite  DataStoreName=closer_point_y_queue  DataStoreElements=closer_point_y_queue  EnableIndexing=on  NumberOfDimensions=2  IndexOptions=Index vector (port),Index vector (dialog)  Indices=1,1  OutputSizes=1,1
  Data Store Write2 : DataStoreWrite  DataStoreName=delta_angle_queue  DataStoreElements=delta_angle_queue  EnableIndexing=on  NumberOfDimensions=2  IndexOptions=Index vector (port),Index vector (dialog)  Indices=1,1  OutputSizes=1,1
  Data Store Write3 : DataStoreWrite  DataStoreName=closer_point_index_queue  DataStoreElements=closer_point_index_queue  EnableIndexing=on  NumberOfDimensions=2  IndexOptions=Index vector (port),Index vector (dialog)  Indices=1,1  OutputSizes=1,1
  Data Store Write4 : DataStoreWrite  DataStoreName=near_lateral_offset_queue  DataStoreElements=near_lateral_offset_queue  EnableIndexing=on  NumberOfDimensions=2  IndexOptions=Index vector (port),Index vector (dialog)  Indices=1,1  OutputSizes=1,1
  Data Store Write5 : DataStoreWrite  DataStoreName=valid_queue_length  IndexOptions=Index vector (dialog)  Indices=1  OutputSizes=1
  Data Store Write6 : DataStoreWrite  DataStoreName=closer_point_curvature_queue  DataStoreElements=closer_point_curvature_queue  EnableIndexing=on  NumberOfDimensions=2  IndexOptions=Index vector (port),Index vector (dialog)  Indices=1,1  OutputSizes=1,1
  Data Store Write7 : DataStoreWrite  DataStoreName=min_delta_angle  IndexOptions=Index vector (dialog)  Indices=1  OutputSizes=1
  Data Store Write9 : DataStoreWrite  DataStoreName=closest_distance  IndexOptions=Index vector (dialog)  Indices=1  OutputSizes=1
  Selector1 : Selector  Description=获取参考轨迹起点、倒数第二个点的y坐标。  IndexOptions=Index vector (port)  Indices=[1 3]  OutputSizes=1
  Selector2 : Selector  Description=获取参考轨迹起点、倒数第二个点的x坐标。  IndexOptions=Index vector (port)  Indices=[1 3]  OutputSizes=1
  Selector3 : Selector  Description=获取参考轨迹起点的横摆角。  IndexOptions=Index vector (port)  Indices=[1 3]  OutputSizes=1
  Selector4 : Selector  Description=获取参考轨迹倒数第二点的横摆角。  IndexOptions=Index vector (port)  Indices=[1 3]  OutputSizes=1
  Selector5 : Selector  Description=获取参考轨迹起点的x坐标。  IndexOptions=Index vector (port)  Indices=[1 3]  OutputSizes=1
  Selector6 : Selector  Description=获取参考轨迹起点的y坐标。  IndexOptions=Index vector (port)  Indices=[1 3]  OutputSizes=1
  Selector7 : Selector  Description=获取参考轨迹倒数第二点的x坐标。  IndexOptions=Index vector (port)  Indices=[1 3]  OutputSizes=1
  Selector8 : Selector  Description=获取参考轨迹倒数第二点的y坐标。  IndexOptions=Index vector (port)  Indices=[1 3]  OutputSizes=1
  Selector9 : Selector  Description=获取参考轨迹起点、倒数第二个点的曲率。  IndexOptions=Index vector (port)  Indices=[1 3]  OutputSizes=1
  Subtract : Sum  Inputs=+-
  Subtract1 : Sum  Inputs=+-
  Subtract2 : Sum  Description=获取参考轨迹倒数第二个路点索引，将倒数第一个路点留给控制预瞄。  Inputs=+-
  Subtract3 : Sum  Description=获取参考轨迹倒数第二个路点索引，将倒数第一个路点留给控制预瞄。  Inputs=+-
  Two_Point_Distance1_Calculate : ModelReference  Description=计算车辆当前点与参考轨迹上第一个路点的距离。  ModelNameDialog=Two_point_distance_calculate.slx  SimulationMode=Normal  ModelReferenceVersion=4.61
  Two_Point_Distance2_Calculate : ModelReference  Description=计算车辆当前点与参考轨迹上倒数第二个路点的距离。  ModelNameDialog=Two_point_distance_calculate.slx  SimulationMode=Normal  ModelReferenceVersion=4.61
  Vector Concatenate : Concatenate
  Vector Concatenate2 : Concatenate
  Vector Concatenate4 : Concatenate
  loop_times : Outport  Description=循环次数，自然数，无量纲。  OutDataTypeStr=int32
  wires:
  Constant1/1 -> Data Store Write/2
  In Bus Element6/1 -> Selector2/1
  In Bus Element1/1 -> Subtract2/1
  Constant2/1 -> Vector Concatenate/1
  Selector2/1 -> Data Store Write/1
  Selector1/1 -> Data Store Write1/1
  In Bus Element2/1 -> Selector1/1
  Constant4/1 -> Data Store Write1/2
  In Bus Element5/1 -> Selector3/1
  Constant6/1 -> Selector3/2
  In Bus Element4/1 -> Subtract/1
  Selector3/1 -> Subtract/2
  Selector4/1 -> Subtract1/2
  In Bus Element7/1 -> Subtract1/1
  In Bus Element8/1 -> Selector4/1
  Custom_Mod1/1 -> Abs/1  "specific_range_delta_angle1"
  Custom_Mod2/1 -> Abs1/1  "specific_range_delta_angle2"
  Constant14/1 -> Data Store Write2/2
  Vector Concatenate2/1 -> Data Store Write2/1
  Constant16/1 -> Data Store Write3/2
  [first_and_next_to_last_point_index] -> Data Store Write3/1
  Constant19/1 -> Selector5/2
  In Bus Element11/1 -> Selector5/1
  In Bus Element12/1 -> Selector6/1
  Constant20/1 -> Selector6/2
  Selector6/1 -> Two_Point_Distance1_Calculate/4
  Selector5/1 -> Two_Point_Distance1_Calculate/3
  In Bus Element13/1 -> Two_Point_Distance1_Calculate/1
  In Bus Element14/1 -> Two_Point_Distance1_Calculate/2
  In Bus Element17/1 -> Two_Point_Distance2_Calculate/2
  In Bus Element18/1 -> Two_Point_Distance2_Calculate/1
  Selector7/1 -> Two_Point_Distance2_Calculate/3
  Selector8/1 -> Two_Point_Distance2_Calculate/4
  In Bus Element16/1 -> Selector8/1
  In Bus Element15/1 -> Selector7/1
  Vector Concatenate4/1 -> Data Store Write4/1
  Constant22/1 -> Data Store Write4/2
  Two_Point_Distance1_Calculate/1 -> Data Store Write9/1, Vector Concatenate4/1  "specific_near_lateral_offset1"
  Two_Point_Distance2_Calculate/1 -> Vector Concatenate4/2  "specific_near_lateral_offset2"
  Constant8/1 -> Custom_Mod1/2
  Constant9/1 -> Custom_Mod1/4
  Constant7/1 -> Custom_Mod1/3
  Constant24/1 -> Custom_Mod2/3
  Constant26/1 -> Custom_Mod2/4
  Constant25/1 -> Custom_Mod2/2
  Subtract/1 -> Custom_Mod1/1  "temp_delta_angle1"
  Subtract1/1 -> Custom_Mod2/1  "temp_delta_angle2"
  Constant11/1 -> Subtract2/2
  Constant23/1 -> Data Store Write5/1
  Abs1/1 -> Vector Concatenate2/2
  Abs/1 -> Data Store Write7/1, Vector Concatenate2/1
  Constant3/1 -> Data Store Write6/2
  In Bus Element3/1 -> Selector9/1
  Selector9/1 -> Data Store Write6/1
  Subtract2/1 -> [next_to_last_point_index]
  [next_to_last_point_index] -> Selector4/2
  Vector Concatenate/1 -> [first_and_next_to_last_point_index]
  [next_to_last_point_index] -> Vector Concatenate/2
  [first_and_next_to_last_point_index] -> Selector2/2
  [first_and_next_to_last_point_index] -> Selector1/2
  [first_and_next_to_last_point_index] -> Selector9/2
  [next_to_last_point_index] -> Selector7/2
  [next_to_last_point_index] -> Selector8/2
  Subtract3/1 -> loop_times/1
  Constant5/1 -> Subtract3/2
  In Bus Element9/1 -> Subtract3/1

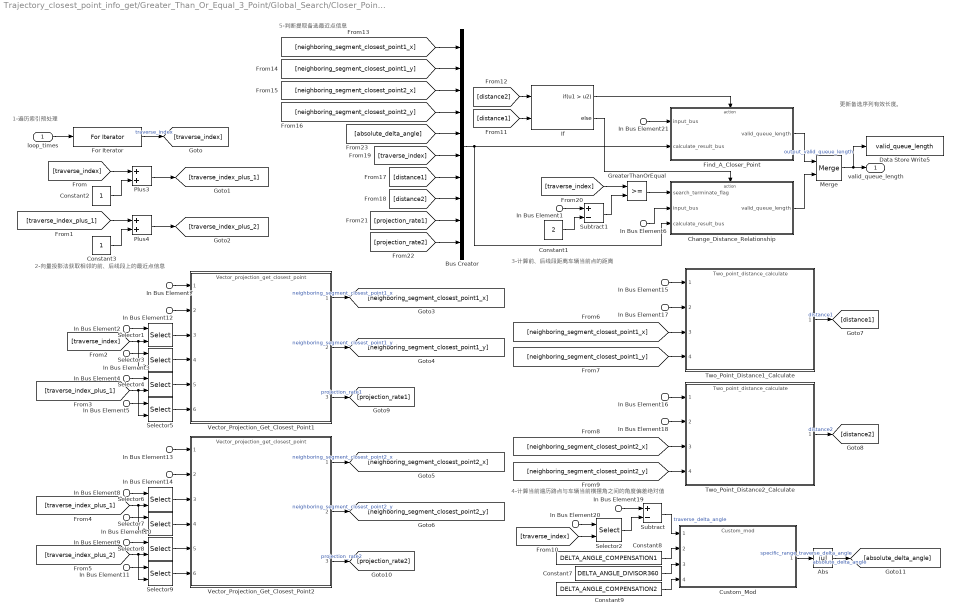
== system Trajectory_closest_point_info_get/Greater_Than_Or_Equal_3_Point/Global_Search/Closer_Point_Queue_Search_Loop ==
  note: 更新备选序列有效长度。
  note: 5-判断提取备选最近点信息
  note: 4-计算当前遍历路点与车辆当前横摆角之间的角度偏差绝对值
  note: 3-计算前、后线段距离车辆当前点的距离
  note: 2-向量投影法获取相邻的前、后线段上的最近点信息
  note: 1-遍历索引预处理
  loop_times : Inport  Description=循环次数，自然数，无量纲。  OutDataTypeStr=int32  Interpolate=off
  In Bus Element6 : Inport  Port=2  PortName=input_bus
  In Bus Element21 : Inport  Port=2  PortName=input_bus
  In Bus Element{2,4,8..9} (4 alike) : Inport  Port=2  PortName=input_bus  Element=trajectory_x
  In Bus Element{3,5,10..11} (4 alike) : Inport  Port=2  PortName=input_bus  Element=trajectory_y
  In Bus Element{7,13,15..16} (4 alike) : Inport  Port=2  PortName=input_bus  Element=current_point_x
  In Bus Element{12,14,17..18} (4 alike) : Inport  Port=2  PortName=input_bus  Element=current_point_y
  In Bus Element19 : Inport  Port=2  PortName=input_bus  Element=current_point_yaw_angle
  In Bus Element20 : Inport  Port=2  PortName=input_bus  Element=trajectory_yaw_angle
  In Bus Element1 : Inport  Port=2  PortName=input_bus  Element=way_point_number
  Abs : Abs
  Bus Creator : BusCreator  Inputs=10
  Change_Distance_Relationship : Subsystem  Description=不满足距离关系条件时，将距离关系转移标志设置为false，等待下一个满足条件的路点。  TreatAsAtomicUnit=on
  Constant1 : Constant  Value=2  OutDataTypeStr=int32  SampleTime=-1
  Constant2 : Constant  OutDataTypeStr=int32  SampleTime=-1
  Constant3 : Constant  OutDataTypeStr=int32  SampleTime=-1
  Constant7 : Constant  Value=DELTA_ANGLE_DIVISOR360  OutDataTypeStr=double  SampleTime=-1
  Constant8 : Constant  Value=DELTA_ANGLE_COMPENSATION1  OutDataTypeStr=double  SampleTime=-1
  Constant9 : Constant  Value=DELTA_ANGLE_COMPENSATION2  OutDataTypeStr=double  SampleTime=-1
  Custom_Mod : ModelReference  Description=对当前车辆横摆角与参考轨迹当前遍历路点横摆角偏差取模到-180~180度范围内。  ModelNameDialog=Custom_mod  SimulationMode=Normal  ModelReferenceVersion=4.78
  Data Store Write5 : DataStoreWrite  DataStoreName=valid_queue_length  IndexOptions=Index vector (dialog)  Indices=1  OutputSizes=1
  Find_A_Closer_Point : Subsystem  Description=当出现后一个线段到当前点的距离大于前一个线段时，说明前一个线段到当前点的最近点是一个备选参考路径最近点。  TreatAsAtomicUnit=on
  For Iterator : ForIterator  ResetStates=reset  IterationSource=external
  GreaterThanOrEqual : RelationalOperator  OutDataTypeStr=boolean  RndMeth=Simplest
  If : If  NumInputs=2  IfExpression=u1 > u2
  Merge : Merge
  Plus3 : Sum  Description=遍历索引加1，代表当前遍历路点的下一个路点。
  Plus4 : Sum  Description=遍历索引加1以后再加1，代表当前遍历路点的下下个路点。
  Selector1 : Selector  Description=获取当前遍历路点的x坐标。  IndexOptions=Index vector (port)  Indices=[1 3]  OutputSizes=1
  Selector2 : Selector  Description=获取参考轨迹当前遍历路点处的横摆角。  IndexOptions=Index vector (port)  Indices=[1 3]  OutputSizes=1
  Selector3 : Selector  Description=获取当前遍历路点的y坐标。  IndexOptions=Index vector (port)  Indices=[1 3]  OutputSizes=1
  Selector4 : Selector  Description=获取当前遍历路点的下一个路点的x坐标。  IndexOptions=Index vector (port)  Indices=[1 3]  OutputSizes=1
  Selector5 : Selector  Description=获取当前遍历路点的下一个路点的y坐标。  IndexOptions=Index vector (port)  Indices=[1 3]  OutputSizes=1
  Selector6 : Selector  Description=获取当前遍历路点的下一个路点的x坐标。  IndexOptions=Index vector (port)  Indices=[1 3]  OutputSizes=1
  Selector7 : Selector  Description=获取当前遍历路点的下一个路点的y坐标。  IndexOptions=Index vector (port)  Indices=[1 3]  OutputSizes=1
  Selector8 : Selector  Description=获取当前遍历路点的下下个路点的x坐标。  IndexOptions=Index vector (port)  Indices=[1 3]  OutputSizes=1
  Selector9 : Selector  Description=获取当前遍历路点的下下个路点的y坐标。  IndexOptions=Index vector (port)  Indices=[1 3]  OutputSizes=1
  Subtract : Sum  Description=计算当前车辆横摆角与参考轨迹当前遍历路点横摆角的差值。  Inputs=+-
  Subtract1 : Sum  Inputs=+-
  Two_Point_Distance1_Calculate : ModelReference  Description=计算车辆当前点与参考轨迹上当前遍历路点和下一个路点所组成的前一个路段的最近点的距离1。  ModelNameDialog=Two_point_distance_calculate.slx  SimulationMode=Normal  ModelReferenceVersion=4.61
  Two_Point_Distance2_Calculate : ModelReference  Description=计算车辆当前点与参考轨迹上当前遍历路点的下一个路点和下下个路点所组成的后一个路段的最近点的距离2。  ModelNameDialog=Two_point_distance_calculate.slx  SimulationMode=Normal  ModelReferenceVersion=4.61
  Vector_Projection_Get_Closest_Point1 : ModelReference  Description=向量投影法获取当前遍历路点与下一个路点之间的最近点1。  ModelNameDialog=Vector_projection_get_closest_point.slx  SimulationMode=Normal  ModelReferenceVersion=4.54
  Vector_Projection_Get_Closest_Point2 : ModelReference  Description=向量投影法获取当前遍历路点的下一个路点与下下个路点之间的最近点2。  ModelNameDialog=Vector_projection_get_closest_point.slx  SimulationMode=Normal  ModelReferenceVersion=4.54
  valid_queue_length : Outport  Description=备选序列有效长度，自然数，无量纲。  OutDataTypeStr=int32
  wires:
  loop_times/1 -> For Iterator/1
  Plus3/1 -> [traverse_index_plus_1]
  Constant2/1 -> Plus3/2
  Constant3/1 -> Plus4/2
  [traverse_index] -> Plus3/1
  Plus4/1 -> [traverse_index_plus_2]
  [traverse_index_plus_1] -> Plus4/1
  For Iterator/1 -> [traverse_index]  "traverse_index"
  Vector_Projection_Get_Closest_Point1/3 -> [projection_rate1]  "projection_rate1"
  Selector5/1 -> Vector_Projection_Get_Closest_Point1/6
  [traverse_index_plus_2] -> Selector8/2, Selector9/2
  Vector_Projection_Get_Closest_Point1/1 -> [neighboring_segment_closest_point1_x]  "neighboring_segment_closest_point1_x"
  Selector8/1 -> Vector_Projection_Get_Closest_Point2/5
  [traverse_index_plus_1] -> Selector7/2, Selector6/2
  In Bus Element8/1 -> Selector6/1
  In Bus Element9/1 -> Selector8/1
  Selector7/1 -> Vector_Projection_Get_Closest_Point2/4
  [traverse_index_plus_1] -> Selector5/2, Selector4/2
  [traverse_index] -> Selector1/2, Selector3/2
  Selector9/1 -> Vector_Projection_Get_Closest_Point2/6
  In Bus Element14/1 -> Vector_Projection_Get_Closest_Point2/2
  In Bus Element4/1 -> Selector4/1
  In Bus Element2/1 -> Selector1/1
  Vector_Projection_Get_Closest_Point2/1 -> [neighboring_segment_closest_point2_x]  "neighboring_segment_closest_point2_x"
  In Bus Element13/1 -> Vector_Projection_Get_Closest_Point2/1
  In Bus Element11/1 -> Selector9/1
  Selector3/1 -> Vector_Projection_Get_Closest_Point1/4
  In Bus Element3/1 -> Selector3/1
  Vector_Projection_Get_Closest_Point1/2 -> [neighboring_segment_closest_point1_y]  "neighboring_segment_closest_point1_y"
  In Bus Element10/1 -> Selector7/1
  Vector_Projection_Get_Closest_Point2/2 -> [neighboring_segment_closest_point2_y]  "neighboring_segment_closest_point2_y"
  Selector1/1 -> Vector_Projection_Get_Closest_Point1/3
  Selector4/1 -> Vector_Projection_Get_Closest_Point1/5
  Selector6/1 -> Vector_Projection_Get_Closest_Point2/3
  In Bus Element5/1 -> Selector5/1
  In Bus Element12/1 -> Vector_Projection_Get_Closest_Point1/2
  In Bus Element7/1 -> Vector_Projection_Get_Closest_Point1/1
  Vector_Projection_Get_Closest_Point2/3 -> [projection_rate2]  "projection_rate2"
  Two_Point_Distance1_Calculate/1 -> [distance1]  "distance1"
  Two_Point_Distance2_Calculate/1 -> [distance2]  "distance2"
  In Bus Element17/1 -> Two_Point_Distance1_Calculate/2
  In Bus Element18/1 -> Two_Point_Distance2_Calculate/2
  [neighboring_segment_closest_point2_x] -> Two_Point_Distance2_Calculate/3
  [neighboring_segment_closest_point2_y] -> Two_Point_Distance2_Calculate/4
  [neighboring_segment_closest_point1_y] -> Two_Point_Distance1_Calculate/4
  In Bus Element16/1 -> Two_Point_Distance2_Calculate/1
  [neighboring_segment_closest_point1_x] -> Two_Point_Distance1_Calculate/3
  In Bus Element15/1 -> Two_Point_Distance1_Calculate/1
  Selector2/1 -> Subtract/2
  Subtract/1 -> Custom_Mod/1  "traverse_delta_angle"
  [traverse_index] -> Selector2/2
  Constant8/1 -> Custom_Mod/2
  In Bus Element19/1 -> Subtract/1
  Constant9/1 -> Custom_Mod/4
  In Bus Element20/1 -> Selector2/1
  Constant7/1 -> Custom_Mod/3
  Custom_Mod/1 -> Abs/1  "specific_range_traverse_delta_angle"
  [distance2] -> If/1
  [distance1] -> If/2
  If/1 -> Find_A_Closer_Point/Action
  [neighboring_segment_closest_point1_x] -> Bus Creator/1
  [neighboring_segment_closest_point1_y] -> Bus Creator/2
  [neighboring_segment_closest_point2_x] -> Bus Creator/3
  [neighboring_segment_closest_point2_y] -> Bus Creator/4
  [traverse_index] -> Bus Creator/6
  [distance1] -> Bus Creator/7
  [distance2] -> Bus Creator/8
  Abs/1 -> [absolute_delta_angle]  "absolute_delta_angle"
  Bus Creator/1 -> Find_A_Closer_Point/2(calculate_result_bus), Change_Distance_Relationship/3(calculate_result_bus)
  If/2 -> Change_Distance_Relationship/Action
  In Bus Element1/1 -> Subtract1/1
  Constant1/1 -> Subtract1/2
  [traverse_index] -> GreaterThanOrEqual/1
  Subtract1/1 -> GreaterThanOrEqual/2
  GreaterThanOrEqual/1 -> Change_Distance_Relationship/1(search_terminate_flag)
  Merge/1 -> valid_queue_length/1, Data Store Write5/1  "output_valid_queue_length"
  [projection_rate2] -> Bus Creator/10
  [projection_rate1] -> Bus Creator/9
  In Bus Element6/1 -> Change_Distance_Relationship/2(input_bus)
  In Bus Element21/1 -> Find_A_Closer_Point/1(input_bus)
  [absolute_delta_angle] -> Bus Creator/5
  Find_A_Closer_Point/1(valid_queue_length) -> Merge/1
  Change_Distance_Relationship/1(valid_queue_length) -> Merge/2

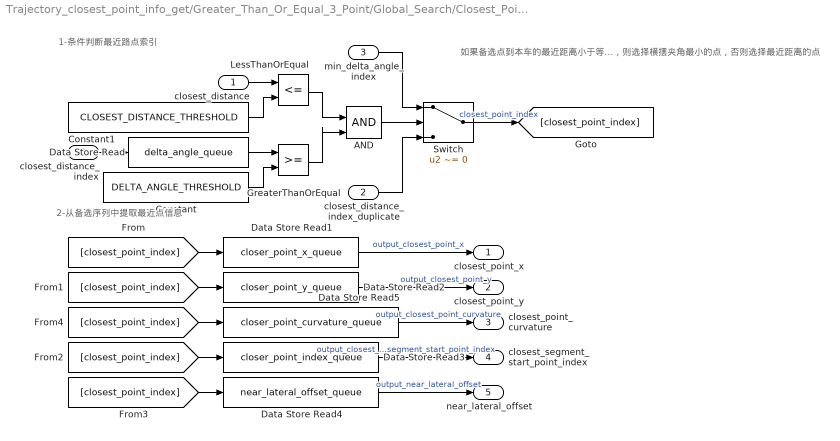
== system Trajectory_closest_point_info_get/Greater_Than_Or_Equal_3_Point/Global_Search/Closest_Point_Get ==
  note: 2-从备选序列中提取最近点信息
  note: 1-条件判断最近路点索引
  note: 如果备选点到本车的最近距离小于等于阈值，且最近距离的点的横摆夹角大于等于90度，则选择横摆夹角最小的点，否则选择最近距离的点
  closest_distance : Inport  Description=备选最近点序列中与车辆当前点之间的最近距离，正实数，m。  OutDataTypeStr=double
  closest_distance_index : Inport  Description=备选最近点序列中与车辆当前点之间的距离最近的路点索引，自然数，无量纲。  Port=2  OutDataTypeStr=int32
  min_delta_angle_index : Inport  Description=备选最近点序列中与当前车辆横摆角偏差最小的路点索引，自然数，无量纲。  Port=3  OutDataTypeStr=int32
  AND : Logic  IconShape=distinctive  AllPortsSameDT=off  OutDataTypeStr=boolean
  Constant : Constant  Value=DELTA_ANGLE_THRESHOLD  OutDataTypeStr=double  SampleTime=-1
  Constant1 : Constant  Value=CLOSEST_DISTANCE_THRESHOLD  OutDataTypeStr=double  SampleTime=-1
  Data Store Read : DataStoreRead  DataStoreName=delta_angle_queue  DataStoreElements=delta_angle_queue  EnableIndexing=on  NumberOfDimensions=2  IndexOptions=Index vector (port),Index vector (dialog)  Indices=1,1  OutputSizes=1,1
  Data Store Read1 : DataStoreRead  DataStoreName=closer_point_x_queue  DataStoreElements=closer_point_x_queue  EnableIndexing=on  NumberOfDimensions=2  IndexOptions=Index vector (port),Index vector (dialog)  Indices=1,1  OutputSizes=1,1
  Data Store Read2 : DataStoreRead  DataStoreName=closer_point_y_queue  DataStoreElements=closer_point_y_queue  EnableIndexing=on  NumberOfDimensions=2  IndexOptions=Index vector (port),Index vector (dialog)  Indices=1,1  OutputSizes=1,1
  Data Store Read3 : DataStoreRead  DataStoreName=closer_point_index_queue  DataStoreElements=closer_point_index_queue  EnableIndexing=on  NumberOfDimensions=2  IndexOptions=Index vector (port),Index vector (dialog)  Indices=1,1  OutputSizes=1,1
  Data Store Read4 : DataStoreRead  DataStoreName=near_lateral_offset_queue  DataStoreElements=near_lateral_offset_queue  EnableIndexing=on  NumberOfDimensions=2  IndexOptions=Index vector (port),Index vector (dialog)  Indices=1,1  OutputSizes=1,1
  Data Store Read5 : DataStoreRead  DataStoreName=closer_point_curvature_queue  DataStoreElements=closer_point_curvature_queue  EnableIndexing=on  NumberOfDimensions=2  IndexOptions=Index vector (port),Index vector (dialog)  Indices=1,1  OutputSizes=1,1
  GreaterThanOrEqual : RelationalOperator  OutDataTypeStr=boolean  RndMeth=Simplest
  LessThanOrEqual : RelationalOperator  Operator=<=  OutDataTypeStr=boolean  RndMeth=Simplest
  Switch : Switch  Description=如果备选点到本车的最近距离小于等于阈值，且最近距离的点的横摆夹角大于等于90度，则选择横摆夹角最小的点，否则选择最近距离的点  Criteria=u2 ~= 0
  closest_distance_index_duplicate : InportShadow  Description=备选最近点序列中与车辆当前点之间的距离最近的路点索引，自然数，无量纲。  Port=2  OutDataTypeStr=int32
  closest_point_x : Outport  Description=最近点x坐标，实数，m。  OutDataTypeStr=double
  closest_point_y : Outport  Description=最近点y坐标，实数，m。  Port=2  OutDataTypeStr=double
  closest_point_curvature : Outport  Description=最近点曲率，实数，1/m。  Port=3  OutDataTypeStr=double
  closest_segment_start_point_index : Outport  Description=最近路点线段起始点索引，自然数，无量纲。  Port=4  OutDataTypeStr=int32
  near_lateral_offset : Outport  Description=最近处横向偏差，实数，m。  Port=5  OutDataTypeStr=double
  wires:
  closest_distance_index/1 -> Data Store Read/1
  Data Store Read/1 -> GreaterThanOrEqual/1
  Constant/1 -> GreaterThanOrEqual/2
  closest_distance/1 -> LessThanOrEqual/1
  Constant1/1 -> LessThanOrEqual/2
  LessThanOrEqual/1 -> AND/1
  GreaterThanOrEqual/1 -> AND/2
  AND/1 -> Switch/2
  min_delta_angle_index/1 -> Switch/1
  closest_distance_index_duplicate/1 -> Switch/3
  Switch/1 -> [closest_point_index]  "closest_point_index"
  [closest_point_index] -> Data Store Read1/1
  Data Store Read1/1 -> closest_point_x/1  "output_closest_point_x"
  [closest_point_index] -> Data Store Read2/1
  Data Store Read2/1 -> closest_point_y/1  "output_closest_point_y"
  [closest_point_index] -> Data Store Read3/1
  Data Store Read3/1 -> closest_segment_start_point_index/1  "output_closest_segment_start_point_index"
  [closest_point_index] -> Data Store Read4/1
  Data Store Read4/1 -> near_lateral_offset/1  "output_near_lateral_offset"
  [closest_point_index] -> Data Store Read5/1
  Data Store Read5/1 -> closest_point_curvature/1  "output_closest_point_curvature"

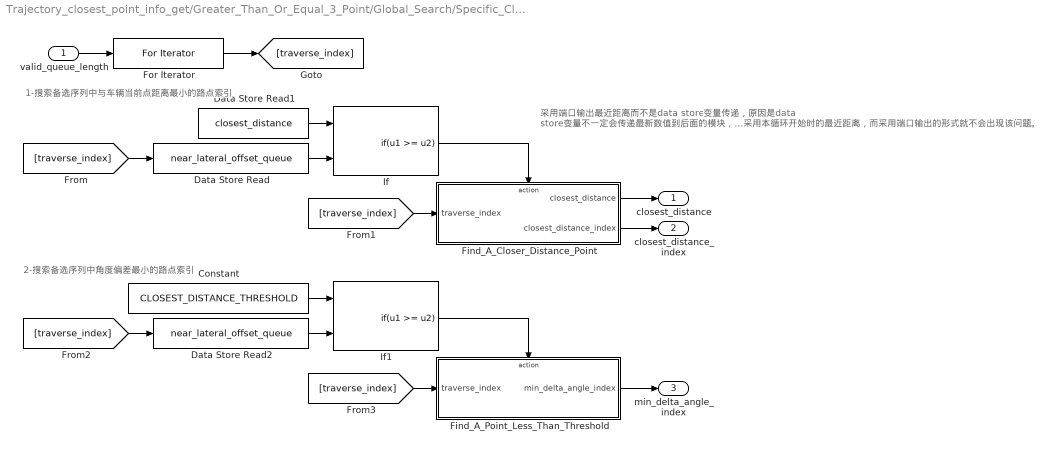
== system Trajectory_closest_point_info_get/Greater_Than_Or_Equal_3_Point/Global_Search/Specific_Closest_Point_Search_Loop ==
  note: 1-搜索备选序列中与车辆当前点距离最小的路点索引
  note: 2-搜索备选序列中角度偏差最小的路点索引
  note: 采用端口输出最近距离而不是data store变量传递，原因是data store变量不一定会传递最新数值到后面的模块，比如只传递采用本循环开始时的最近距离，而采用端口输出的形式就不会出现该问题。
  valid_queue_length : Inport  Description=备选序列有效长度，自然数，无量纲。  OutDataTypeStr=int32  Interpolate=off
  Constant : Constant  Value=CLOSEST_DISTANCE_THRESHOLD  OutDataTypeStr=double  SampleTime=-1
  Data Store Read : DataStoreRead  DataStoreName=near_lateral_offset_queue  DataStoreElements=near_lateral_offset_queue  EnableIndexing=on  NumberOfDimensions=2  IndexOptions=Index vector (port),Index vector (dialog)  Indices=1,1  OutputSizes=1,1
  Data Store Read1 : DataStoreRead  DataStoreName=closest_distance  IndexOptions=Index vector (dialog)  Indices=1  OutputSizes=1
  Data Store Read2 : DataStoreRead  DataStoreName=near_lateral_offset_queue  DataStoreElements=near_lateral_offset_queue  EnableIndexing=on  NumberOfDimensions=2  IndexOptions=Index vector (port),Index vector (dialog)  Indices=1,1  OutputSizes=1,1
  Find_A_Closer_Distance_Point : Subsystem  Description=找到一个与本车距离更近的点。  TreatAsAtomicUnit=on
  Find_A_Point_Less_Than_Threshold : Subsystem  Description=找到一个小于距离阈值的点。  TreatAsAtomicUnit=on
  For Iterator : ForIterator  ResetStates=reset  IterationSource=external
  If : If  NumInputs=2  IfExpression=u1 >= u2  ShowElse=off
  If1 : If  NumInputs=2  IfExpression=u1 >= u2  ShowElse=off
  closest_distance : Outport  Description=备选最近点序列中与车辆当前点之间的最近距离，正实数，m。  OutDataTypeStr=double
  closest_distance_index : Outport  Description=备选最近点序列中与车辆当前点之间的距离最近的路点索引，自然数，无量纲。  Port=2  OutDataTypeStr=int32
  min_delta_angle_index : Outport  Description=备选最近点序列中与当前车辆横摆角偏差最小的路点索引，自然数，无量纲。  Port=3  OutDataTypeStr=int32
  wires:
  For Iterator/1 -> [traverse_index]
  valid_queue_length/1 -> For Iterator/1
  Data Store Read1/1 -> If/1
  Data Store Read/1 -> If/2
  [traverse_index] -> Data Store Read/1
  If/1 -> Find_A_Closer_Distance_Point/Action
  [traverse_index] -> Find_A_Closer_Distance_Point/1(traverse_index)
  [traverse_index] -> Data Store Read2/1
  Data Store Read2/1 -> If1/2
  Constant/1 -> If1/1
  If1/1 -> Find_A_Point_Less_Than_Threshold/Action
  [traverse_index] -> Find_A_Point_Less_Than_Threshold/1(traverse_index)
  Find_A_Point_Less_Than_Threshold/1(min_delta_angle_index) -> min_delta_angle_index/1
  Find_A_Closer_Distance_Point/2(closest_distance_index) -> closest_distance_index/1
  Find_A_Closer_Distance_Point/1(closest_distance) -> closest_distance/1
